simulink model "typical_motor_system_2021a"  (R2021b)
settings: Solver=ode5  StartTime=0.0  StopTime=10.0  FixedStep=1e-4  RelTol=1e-3
settings Model: Creator=wkw  LastModifiedBy=wkw

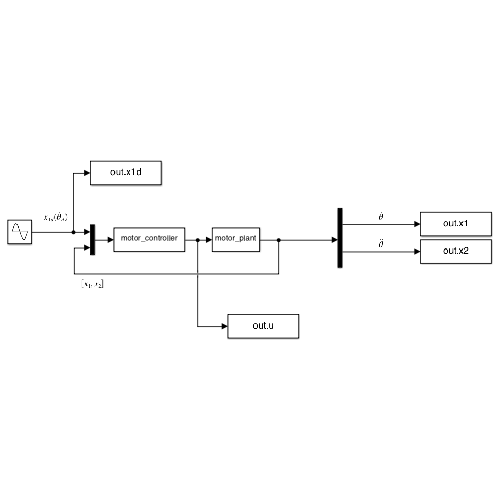
[thumbnail: Simulink's stored preview of the top-level diagram]
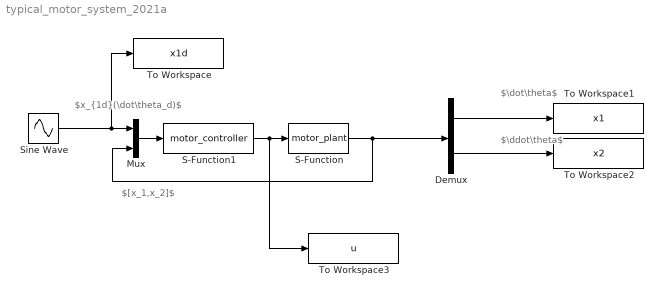
== system typical_motor_system_2021a ==
  note: $\dot\theta$
  note: $[x_1,x_2]$
  note: $x_{1d}(\dot\theta_d)$
  note: $\ddot\theta$
  Demux : Demux  Outputs=2
  Mux : Mux  Inputs=2
  S-Function : S-Function  FunctionName=motor_plant  SFunctionDeploymentMode=off  EnableBusSupport=off
  S-Function1 : S-Function  FunctionName=motor_controller  SFunctionDeploymentMode=off  EnableBusSupport=off
  Sine Wave : Sin  SampleTime=0
  To Workspace : ToWorkspace  VariableName=x1d  SaveFormat=Timeseries  SampleTime=-1
  To Workspace1 : ToWorkspace  VariableName=x1  SaveFormat=Timeseries  SampleTime=-1
  To Workspace2 : ToWorkspace  VariableName=x2  SaveFormat=Timeseries  SampleTime=-1
  To Workspace3 : ToWorkspace  VariableName=u  SaveFormat=Timeseries  SampleTime=-1
  wires:
  Mux/1 -> S-Function1/1
  Sine Wave/1 -> To Workspace/1, Mux/1
  S-Function/1 -> Demux/1, Mux/2
  S-Function1/1 -> To Workspace3/1, S-Function/1
  Demux/1 -> To Workspace1/1
  Demux/2 -> To Workspace2/1
